simulink model "Xe_Model_Redo_June_26"  (R2018a)
settings: Solver=VariableStepAuto  StartTime=0.0  StopTime=5E5+96*60*60  RelTol=1e-3
values from neighbouring files (symbols this model uses):
  A_pipe = pi*r_pipe^2    (= 0.0126676869774)    [Startup_Script.m]
  alpha_FS = 0.517E-16    (= 5.17e-17)    [Startup_Script.m]
  alpha_G_R1 = 0.334E-17    (= 3.34e-18)    [Startup_Script.m]
  alpha_G_R2 = 0.699E-17    (= 6.99e-18)    [Startup_Script.m]
  alpha_G_R3 = 0.669E-17    (= 6.69e-18)    [Startup_Script.m]
  alpha_G_R4 = 0.791E-18    (= 7.91e-19)    [Startup_Script.m]
  D_g = 2.37E-9    (= 2.37e-09)    [Startup_Script.m]
  epsilon = 0.1    [Startup_Script.m]
  eta_b = 1E-4    (= 0.0001)    [Startup_Script.m]
  eta_fs = 1.2E-4    (= 0.00012)    [Startup_Script.m]
  f_cv = 0.004    [Startup_Script.m]
  FS_Mu_A = 4340    [Startup_Script.m]
  FS_Mu_K = 0.084    [Startup_Script.m]
  FS_Mu_MSRE = 0.007027    [Startup_Script.m]
  FS_rho_A = 3.628    [Startup_Script.m]
  FS_rho_B = 0.00066    [Startup_Script.m]
  FS_rho_MSRE = 2082    [Startup_Script.m]
  gamma_i = 0.0293524    [Startup_Script.m]
  gamma_te = 0.0322482    [Startup_Script.m]
  gamma_xe = 0.00257324    [Startup_Script.m]
  h_fc = 1.6    [Startup_Script.m]
  H_Xe_a = 5.713e-13    [Startup_Script.m]
  H_Xe_b = -7.937e-10    [Startup_Script.m]
  H_Xe_c = 2.809e-07    [Startup_Script.m]
  HX_r_Tube = ((0.5-0.042)/2)*2.54E-2    (= 0.0058166)    [Startup_Script.m]
  HX_XS = HX_N_Tubes*(pi*HX_r_Tube^2)    (= 0.0168999490356)    [Startup_Script.m]
  k_b = 1.3806E-23    (= 1.3806e-23)    [Startup_Script.m]
  lambda_i = 2.9306070546251702E-5    (= 2.93060705463e-05)    [Startup_Script.m]
  lambda_te = 0.036481430555786593    (= 0.0364814305558)    [Startup_Script.m]
  lambda_xe = 2.0924e-05    [Startup_Script.m]
  N_FC_R1 = 12    [Startup_Script.m]
  N_FC_R2 = 940    [Startup_Script.m]
  N_FC_R3 = 108    [Startup_Script.m]
  N_FC_R4 = 78    [Startup_Script.m]
  P_pump = 35420    [Startup_Script.m]
  phi0 = 3.98E+17    (= 3.98e+17)    [Startup_Script.m]
  phi_G_R_1 = mean(interp1(phi_G_R,phi_G_phi, linspace(0,r_g_r1)))    [Startup_Script.m]
  phi_G_R_2 = mean(interp1(phi_G_R,phi_G_phi, linspace(r_g_r1,r_g_r2)))    [Startup_Script.m]
  phi_G_R_3 = mean(interp1(phi_G_R,phi_G_phi, linspace(r_g_r2,r_g_r3)))    [Startup_Script.m]
  phi_G_R_4 = mean(interp1(phi_G_R,phi_G_phi, linspace(r_g_r3,r_g_r4)))    [Startup_Script.m]
  Q_strpr = 0.003155    [Startup_Script.m]
  Q_tot = 0.07571    [Startup_Script.m]
  r_b = 0.000254    [Startup_Script.m]
  r_fc = 0.79e-2    (= 0.0079)    [Startup_Script.m]
  r_pipe = (5E-2*2.54)/2    (= 0.0635)    [Startup_Script.m]
  r_xe = 2.16E-10    (= 2.16e-10)    [Startup_Script.m]
  Re_CA = 25800    [Startup_Script.m]
  Re_LH = 1E4    (= 10000)    [Startup_Script.m]
  Re_UH = 1E4    (= 10000)    [Startup_Script.m]
  sig_a_xe = 1.18E-22    (= 1.18e-22)    [Startup_Script.m]
  Sig_f = 0.15    [Startup_Script.m]
  T_CA_0 = T_INLET    (= 907.594444444)    [Startup_Script.m]
  T_FP_0 = T_OUTLET    (= 935.372222222)    [Startup_Script.m]
  T_FS_R_1_0 = mean(interp1(R_fs_m,T_fs_K, linspace(0,r_g_r1)))    [Startup_Script.m]
  T_FS_R_2_0 = mean(interp1(R_fs_m,T_fs_K, linspace(r_g_r1,r_g_r2)))    [Startup_Script.m]
  T_FS_R_3_0 = mean(interp1(R_fs_m,T_fs_K, linspace(r_g_r2,r_g_r3)))    [Startup_Script.m]
  T_FS_R_4_0 = mean(interp1(R_fs_m,T_fs_K, linspace(r_g_r3,r_g_r4)))    [Startup_Script.m]
  T_G_R_1_0 = mean(interp1(R_gr_m,T_gr_K, linspace(0,r_g_r1)))    [Startup_Script.m]
  T_HX_0 = 0.5*(T_OUTLET + T_INLET)    (= 921.483333333)    [Startup_Script.m]
  T_LH_0 = T_INLET    (= 907.594444444)    [Startup_Script.m]
  T_Mes = 928.15    [Startup_Script.m]
  T_P100_0 = T_OUTLET    (= 935.372222222)    [Startup_Script.m]
  T_P101_0 = T_OUTLET    (= 935.372222222)    [Startup_Script.m]
  T_P102_0 = T_INLET    (= 907.594444444)    [Startup_Script.m]
  T_Salt_0 = 900    [Startup_Script.m]
  T_UH_0 = T_OUTLET    (= 935.372222222)    [Startup_Script.m]
  U_FC_R1 = 0.607    [Startup_Script.m]
  U_FC_R2 = 0.183    [Startup_Script.m]
  U_FC_R3 = 0.454    [Startup_Script.m]
  U_FC_R4 = 0.250    (= 0.25)    [Startup_Script.m]
  V_CA_0 = 9.7*cubed_foot_to_cubed_meter    (= 0.274673445)    [Startup_Script.m]
  V_FP_0 = (0.9+3.2)*cubed_foot_to_cubed_meter    (= 0.116099085)    [Startup_Script.m]
  V_HX_0 = 6.1*cubed_foot_to_cubed_meter    (= 0.172732785)    [Startup_Script.m]
  V_LH_0 = 10.0*cubed_foot_to_cubed_meter    (= 0.2831685)    [Startup_Script.m]
  V_P100_0 = 2.1*cubed_foot_to_cubed_meter    (= 0.059465385)    [Startup_Script.m]
  V_P101_0 = 0.8*cubed_foot_to_cubed_meter    (= 0.02265348)    [Startup_Script.m]
  V_P102_0 = 2.2*cubed_foot_to_cubed_meter    (= 0.06229707)    [Startup_Script.m]
  V_R1_0 = V_Core_FS_0 *N_FC_R1/N_FC_tot    (= 0.00753107712766)    [Startup_Script.m]
  V_R2_0 = V_Core_FS_0 *N_FC_R2/N_FC_tot    (= 0.589934375)    [Startup_Script.m]
  V_R3_0 = V_Core_FS_0 *N_FC_R3/N_FC_tot    (= 0.0677796941489)    [Startup_Script.m]
  V_R4_0 = V_Core_FS_0 *N_FC_R4/N_FC_tot    (= 0.0489520013298)    [Startup_Script.m]
  V_UH_0 = 10.5*cubed_foot_to_cubed_meter    (= 0.297326925)    [Startup_Script.m]
undefined symbols (not defined in the file or in its folder): magnitude, V_CA, V_HX, V_P2, V_P3, V_R1, V_R2, V_R3, V_R4, V_UH
libraries: simulink x4, dspindex x4, dspstat3 x4, SignalEditorBlockLib x2
(part 3 of 11)

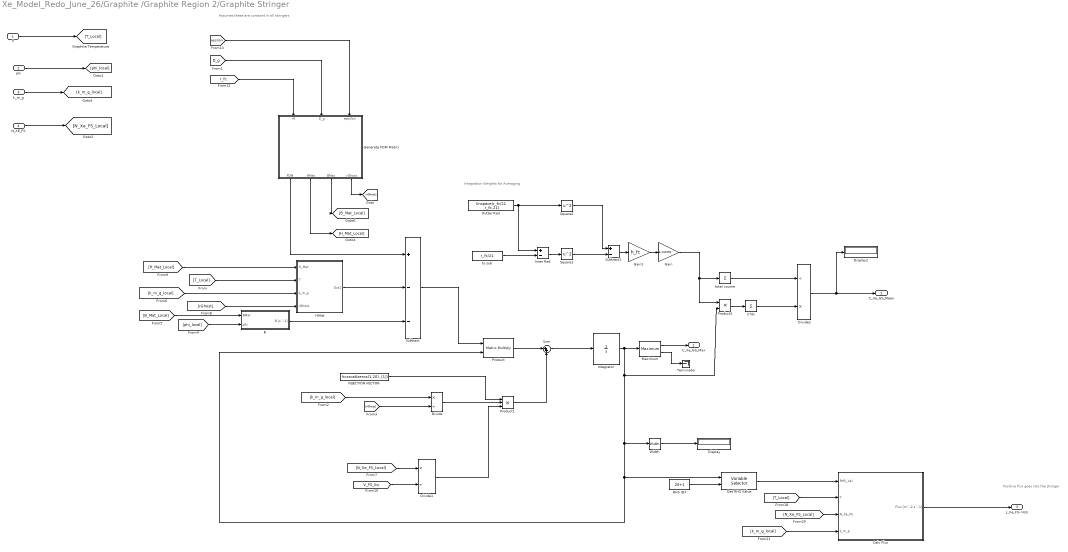
== system Xe_Model_Redo_June_26/Graphite /Graphite Region 2/Graphite Stringer ==
  note: Integration Weights for Averaging
  note: Assumes these are constant in all stringers
  note: Positive flux goes into the stringer
  T : Inport
  phi : Inport  Port=2
  k_m_g : Inport  Port=3
  N_XE_FS : Inport  Port=4
  B : Subsystem
  C*dv : Sum  Inputs=+
  Calc Flux : Subsystem
  Display : Display
  Display2 : Display
  Divide : Product  Inputs=*/
  Divide1 : Product  Inputs=*/
  Divide2 : Product  Inputs=/*
  Gain : Gain  Gain=3.141592
  Gain1 : Gain  Gain=h_fc
  "Generate FDM Matrix " : MATLAB Function  TreatAsAtomicUnit=on
  Get RHS Value : dspindex/Variable Selector  NumInputs=1  rowsOrCols=Rows  IdxMode=Variable  Elements=[1 3]  ZerOneIdxMode=One-based  errmode=Clip Index  FillMode=on  FillValues=0
  HMat : Subsystem
  INJECTION VECTOR : Constant  Value=horzcat(zeros(1,20), [1])
  Inner Rad : Sum  Inputs=+-
  Integrator : Integrator
  Maximum : dspstat3/Maximum  operation=maximum  fcn=Value and Index  indexBase=One  operateOver=Each column  Dimension=1  InputProcessing=Columns as channels (frame based)  reset=None  roiEnable=off  roiType=Rectangles  roiPortion=Entire ROI  roiOutput=Individual statistics for each ROI  roiFlag=off  roundingMode=Floor  overflowMode=off  accumDataTypeStr=Inherit: Same as product output  accumLastDataTypeStr=Inherit: Same as product output
  Outter Rad : Constant  Value=linspace(r_fc/21 ,r_fc,21)
  Product : Product  Multiplication=Matrix(*)
  Product1 : Product  Inputs=3
  Product2 : Product
  RHS IDX : Constant  Value=20+1
  Square1 : Math  Operator=square  SaturateOnIntegerOverflow=on
  Square2 : Math  Operator=square  SaturateOnIntegerOverflow=on
  Subtract : Sum  Inputs=+--
  Subtract1 : Sum  Inputs=+-
  Sum : Sum  Inputs=|++
  Terminator : Terminator
  Width : Width
  to sub : Constant  Value=r_fc/21
  total voume : Sum  Inputs=+
  C_Xe_GS_Max : Outport
  C_Xe_GS_Mean : Outport  Port=2
  J_Xe_FS->GS : Outport  Port=3
  wires:
  Get RHS Value/1 -> Calc Flux/1(RHS_Val)
  Calc Flux/1("Flux [m^-2 s^-1] ") -> J_Xe_FS->GS/1
  HMat/1(Out1) -> Subtract/2
  Maximum/1 -> C_Xe_GS_Max/1
  [rGhost] -> Divide/2
  Divide/1 -> Product1/2
  "Generate FDM Matrix "/1(FDM) -> Subtract/1
  "Generate FDM Matrix "/4(rGhost) -> [rGhost]
  [B_Mat_Local] -> B/1(BMat)
  phi/1 -> [phi_local]
  Subtract/1 -> Product/1
  Divide1/1 -> Product1/3
  Integrator/1 -> Product2/2, Width/1, Product/2, Get RHS Value/1, Maximum/1
  INJECTION VECTOR/1 -> Product1/1
  Product/1 -> Sum/1
  [T_Local] -> HMat/2(T)
  [epsilon] -> "Generate FDM Matrix "/3(epsilon)
  k_m_g/1 -> [k_m_g_local]
  [phi_local] -> B/2(phi)
  [k_m_g_local] -> HMat/3(k_m_g)
  [D_g] -> "Generate FDM Matrix "/2(D_g)
  "Generate FDM Matrix "/3(BMat) -> [B_Mat_Local]
  T/1 -> [T_Local]
  "Generate FDM Matrix "/2(HMat) -> [H_Mat_Local]
  [H_Mat_Local] -> HMat/1(H_Mat)
  [rGhost] -> HMat/4(rGhost)
  [k_m_g_local] -> Divide/1
  [r_fc] -> "Generate FDM Matrix "/1(r0)
  B/1("B [s^-1] ") -> Subtract/3
  Product1/1 -> Sum/2
  Sum/1 -> Integrator/1
  [V_FS_liq] -> Divide1/2
  RHS IDX/1 -> Get RHS Value/2
  [T_Local] -> Calc Flux/2(T)
  N_XE_FS/1 -> [N_Xe_FS_Local]
  [N_Xe_FS_Local] -> Divide1/1
  [k_m_g_local] -> Calc Flux/4(k_m_g)
  [N_Xe_FS_Local] -> Calc Flux/3(N_Xe_FS)
  Width/1 -> Display/1
  Outter Rad/1 -> Inner Rad/1, Square2/1
  Subtract1/1 -> Gain1/1
  Square1/1 -> Subtract1/2
  Square2/1 -> Subtract1/1
  Gain1/1 -> Gain/1
  to sub/1 -> Inner Rad/2
  Inner Rad/1 -> Square1/1
  Gain/1 -> Product2/1, total voume/1
  total voume/1 -> Divide2/1
  Product2/1 -> C*dv/1
  Divide2/1 -> Display2/1, C_Xe_GS_Mean/1
  C*dv/1 -> Divide2/2
  Maximum/2 -> Terminator/1

== system Xe_Model_Redo_June_26/Graphite /Graphite Region 3/Graphite MTC R1 ==
  note: Diemnsionless Numbers
  note: Thermophysical Properties
  T_Salt : Inport
  U_FC [m/s] : Inport  Port=2
  Constant : Constant  Value=0.023
  Constant1 : Constant  Value=0.8
  Constant2 : Constant  Value=0.4
  Density W Scaling : Subsystem
  Display : Display
  Divide : Product  Inputs=*/
  Gain : Gain  Gain=2
  Mass Diffusion Coeffecient [m^2 /s] : Subsystem
  Math Function : Math  Operator=pow  SaturateOnIntegerOverflow=on
  Math Function1 : Math  Operator=pow  SaturateOnIntegerOverflow=on
  Product : Product
  Reynolds Number : Subsystem
  Schmidt Number : Subsystem
  Sherwood Number : Product  Inputs=3
  Viscosity W Scaling : Subsystem
  k_m_g [m/s] : Outport
  wires:
  [D_FS_Local] -> Divide/1
  Constant2/1 -> Math Function1/2
  [r_fc] -> Gain/1
  Constant/1 -> Sherwood Number/1
  Sherwood Number/1 -> Product/1
  [Sc_FC_Local] -> Math Function1/1
  Divide/1 -> Product/2
  Math Function/1 -> Sherwood Number/2
  Constant1/1 -> Math Function/2
  Product/1 -> k_m_g [m/s]/1
  [Re_FC_Local] -> Math Function/1
  Math Function1/1 -> Sherwood Number/3
  Viscosity W Scaling/1(mu [Pa-s]) -> Mass Diffusion Coeffecient [m^2 /s]/1(Mu), [Mu_FS_Local]
  Density W Scaling/1(rho_FS [kg/m^3]) -> [Rho_FS_Local]
  Mass Diffusion Coeffecient [m^2 /s]/1(D [m^2/s]) -> [D_FS_Local]
  T_Salt/1 -> Mass Diffusion Coeffecient [m^2 /s]/2(T_Salt [k]), Density W Scaling/1(T_Salt [k]), Viscosity W Scaling/1(T_Salt [k])
  Schmidt Number/1(Sc) -> [Sc_FC_Local]
  Reynolds Number/1(Re) -> Display/1, [Re_FC_Local]
  U_FC [m/s]/1 -> Reynolds Number/1(Flow_Velocity [m/s])
  [Rho_FS_Local] -> Reynolds Number/2(rho [kg/m^3])
  [Mu_FS_Local] -> Reynolds Number/3(mu [Pa s])
  [Mu_FS_Local] -> Schmidt Number/1(mu [Pa s])
  [Rho_FS_Local] -> Schmidt Number/2(rho [kg/m^3])
  [D_FS_Local] -> Schmidt Number/3(D [m^2/s])
  Gain/1 -> Divide/2

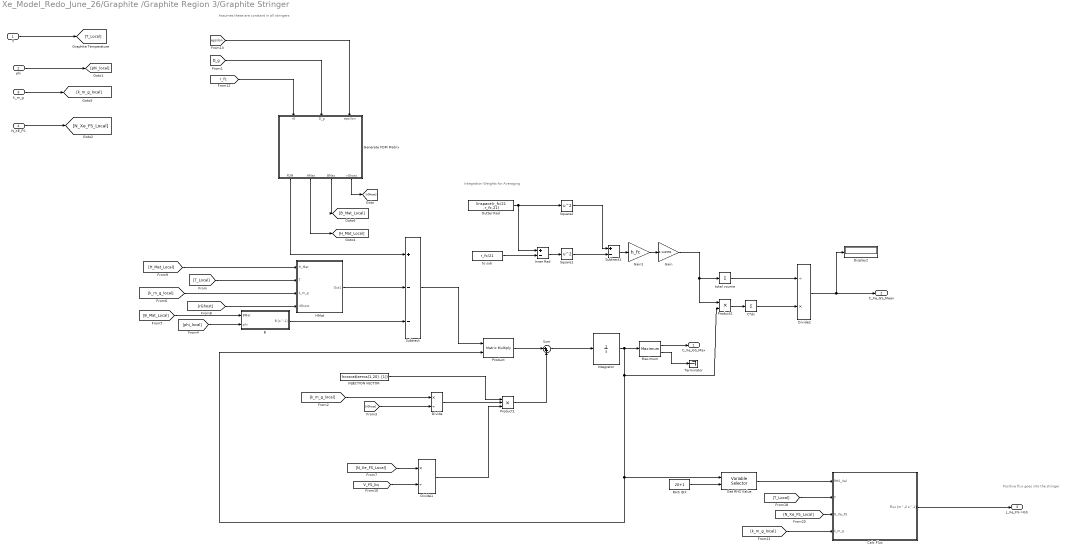
== system Xe_Model_Redo_June_26/Graphite /Graphite Region 3/Graphite Stringer ==
  note: Integration Weights for Averaging
  note: Assumes these are constant in all stringers
  note: Positive flux goes into the stringer
  T : Inport
  phi : Inport  Port=2
  k_m_g : Inport  Port=3
  N_XE_FS : Inport  Port=4
  B : Subsystem
  C*dv : Sum  Inputs=+
  Calc Flux : Subsystem
  Display2 : Display
  Divide : Product  Inputs=*/
  Divide1 : Product  Inputs=*/
  Divide2 : Product  Inputs=/*
  Gain : Gain  Gain=3.141592
  Gain1 : Gain  Gain=h_fc
  "Generate FDM Matrix " : MATLAB Function  TreatAsAtomicUnit=on
  Get RHS Value : dspindex/Variable Selector  NumInputs=1  rowsOrCols=Rows  IdxMode=Variable  Elements=[1 3]  ZerOneIdxMode=One-based  errmode=Clip Index  FillMode=on  FillValues=0
  HMat : Subsystem
  INJECTION VECTOR : Constant  Value=horzcat(zeros(1,20), [1])
  Inner Rad : Sum  Inputs=+-
  Integrator : Integrator
  Maximum : dspstat3/Maximum  operation=maximum  fcn=Value and Index  indexBase=One  operateOver=Each column  Dimension=1  InputProcessing=Columns as channels (frame based)  reset=None  roiEnable=off  roiType=Rectangles  roiPortion=Entire ROI  roiOutput=Individual statistics for each ROI  roiFlag=off  roundingMode=Floor  overflowMode=off  accumDataTypeStr=Inherit: Same as product output  accumLastDataTypeStr=Inherit: Same as product output
  Outter Rad : Constant  Value=linspace(r_fc/21 ,r_fc,21)
  Product : Product  Multiplication=Matrix(*)
  Product1 : Product  Inputs=3
  Product2 : Product
  RHS IDX : Constant  Value=20+1
  Square1 : Math  Operator=square  SaturateOnIntegerOverflow=on
  Square2 : Math  Operator=square  SaturateOnIntegerOverflow=on
  Subtract : Sum  Inputs=+--
  Subtract1 : Sum  Inputs=+-
  Sum : Sum  Inputs=|++
  Terminator : Terminator
  to sub : Constant  Value=r_fc/21
  total voume : Sum  Inputs=+
  C_Xe_GS_Max : Outport
  C_Xe_GS_Mean : Outport  Port=2
  J_Xe_FS->GS : Outport  Port=3
  wires:
  Get RHS Value/1 -> Calc Flux/1(RHS_Val)
  Calc Flux/1("Flux [m^-2 s^-1] ") -> J_Xe_FS->GS/1
  HMat/1(Out1) -> Subtract/2
  Maximum/1 -> C_Xe_GS_Max/1
  [rGhost] -> Divide/2
  Divide/1 -> Product1/2
  "Generate FDM Matrix "/1(FDM) -> Subtract/1
  "Generate FDM Matrix "/4(rGhost) -> [rGhost]
  [B_Mat_Local] -> B/1(BMat)
  phi/1 -> [phi_local]
  Subtract/1 -> Product/1
  Divide1/1 -> Product1/3
  Integrator/1 -> Product2/2, Product/2, Get RHS Value/1, Maximum/1
  INJECTION VECTOR/1 -> Product1/1
  Product/1 -> Sum/1
  [T_Local] -> HMat/2(T)
  [epsilon] -> "Generate FDM Matrix "/3(epsilon)
  k_m_g/1 -> [k_m_g_local]
  [phi_local] -> B/2(phi)
  [k_m_g_local] -> HMat/3(k_m_g)
  [D_g] -> "Generate FDM Matrix "/2(D_g)
  "Generate FDM Matrix "/3(BMat) -> [B_Mat_Local]
  T/1 -> [T_Local]
  "Generate FDM Matrix "/2(HMat) -> [H_Mat_Local]
  [H_Mat_Local] -> HMat/1(H_Mat)
  [rGhost] -> HMat/4(rGhost)
  [k_m_g_local] -> Divide/1
  [r_fc] -> "Generate FDM Matrix "/1(r0)
  B/1("B [s^-1] ") -> Subtract/3
  Product1/1 -> Sum/2
  Sum/1 -> Integrator/1
  [V_FS_liq] -> Divide1/2
  RHS IDX/1 -> Get RHS Value/2
  [T_Local] -> Calc Flux/2(T)
  N_XE_FS/1 -> [N_Xe_FS_Local]
  [N_Xe_FS_Local] -> Divide1/1
  [k_m_g_local] -> Calc Flux/4(k_m_g)
  [N_Xe_FS_Local] -> Calc Flux/3(N_Xe_FS)
  Outter Rad/1 -> Inner Rad/1, Square2/1
  Subtract1/1 -> Gain1/1
  Square1/1 -> Subtract1/2
  Square2/1 -> Subtract1/1
  Gain1/1 -> Gain/1
  to sub/1 -> Inner Rad/2
  Inner Rad/1 -> Square1/1
  Gain/1 -> Product2/1, total voume/1
  total voume/1 -> Divide2/1
  Product2/1 -> C*dv/1
  Divide2/1 -> Display2/1, C_Xe_GS_Mean/1
  C*dv/1 -> Divide2/2
  Maximum/2 -> Terminator/1

== system Xe_Model_Redo_June_26/Graphite /Graphite Region 4/Graphite MTC R1 ==
  note: Diemnsionless Numbers
  note: Thermophysical Properties
  T_Salt : Inport
  U_FC [m/s] : Inport  Port=2
  Constant : Constant  Value=0.023
  Constant1 : Constant  Value=0.8
  Constant2 : Constant  Value=0.4
  Density W Scaling : Subsystem
  Display : Display
  Divide : Product  Inputs=*/
  Gain : Gain  Gain=2
  Mass Diffusion Coeffecient [m^2 /s] : Subsystem
  Math Function : Math  Operator=pow  SaturateOnIntegerOverflow=on
  Math Function1 : Math  Operator=pow  SaturateOnIntegerOverflow=on
  Product : Product
  Reynolds Number : Subsystem
  Schmidt Number : Subsystem
  Sherwood Number : Product  Inputs=3
  Viscosity W Scaling : Subsystem
  k_m_g [m/s] : Outport
  wires:
  [D_FS_Local] -> Divide/1
  Constant2/1 -> Math Function1/2
  [r_fc] -> Gain/1
  Constant/1 -> Sherwood Number/1
  Sherwood Number/1 -> Product/1
  [Sc_FC_Local] -> Math Function1/1
  Divide/1 -> Product/2
  Math Function/1 -> Sherwood Number/2
  Constant1/1 -> Math Function/2
  Product/1 -> k_m_g [m/s]/1
  [Re_FC_Local] -> Math Function/1
  Math Function1/1 -> Sherwood Number/3
  Viscosity W Scaling/1(mu [Pa-s]) -> Mass Diffusion Coeffecient [m^2 /s]/1(Mu), [Mu_FS_Local]
  Density W Scaling/1(rho_FS [kg/m^3]) -> [Rho_FS_Local]
  Mass Diffusion Coeffecient [m^2 /s]/1(D [m^2/s]) -> [D_FS_Local]
  T_Salt/1 -> Mass Diffusion Coeffecient [m^2 /s]/2(T_Salt [k]), Density W Scaling/1(T_Salt [k]), Viscosity W Scaling/1(T_Salt [k])
  Schmidt Number/1(Sc) -> [Sc_FC_Local]
  Reynolds Number/1(Re) -> Display/1, [Re_FC_Local]
  U_FC [m/s]/1 -> Reynolds Number/1(Flow_Velocity [m/s])
  [Rho_FS_Local] -> Reynolds Number/2(rho [kg/m^3])
  [Mu_FS_Local] -> Reynolds Number/3(mu [Pa s])
  [Mu_FS_Local] -> Schmidt Number/1(mu [Pa s])
  [Rho_FS_Local] -> Schmidt Number/2(rho [kg/m^3])
  [D_FS_Local] -> Schmidt Number/3(D [m^2/s])
  Gain/1 -> Divide/2

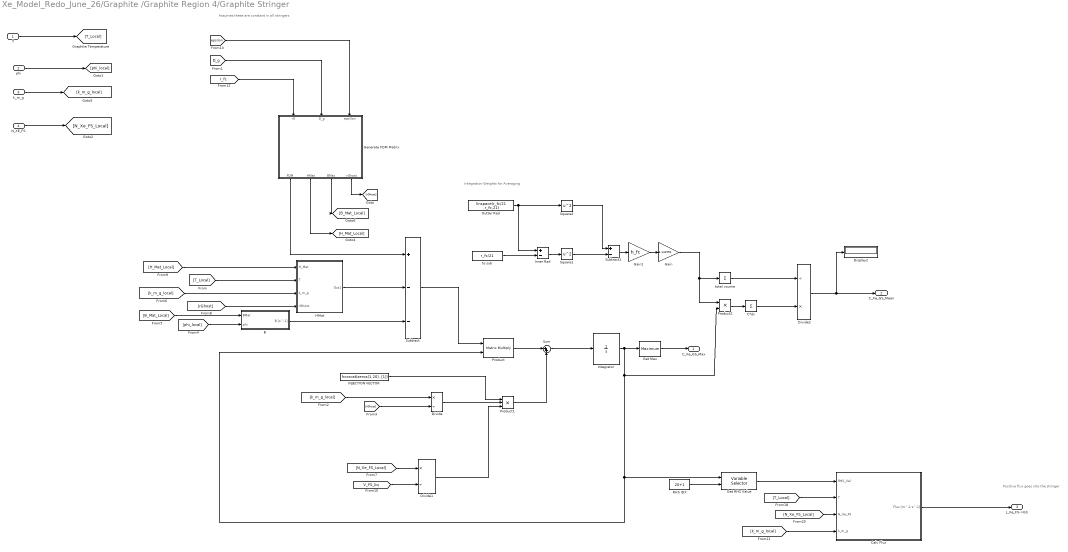
== system Xe_Model_Redo_June_26/Graphite /Graphite Region 4/Graphite Stringer ==
  note: Integration Weights for Averaging
  note: Assumes these are constant in all stringers
  note: Positive flux goes into the stringer
  T : Inport
  phi : Inport  Port=2
  k_m_g : Inport  Port=3
  N_XE_FS : Inport  Port=4
  B : Subsystem
  C*dv : Sum  Inputs=+
  Calc Flux : Subsystem
  Display2 : Display
  Divide : Product  Inputs=*/
  Divide1 : Product  Inputs=*/
  Divide2 : Product  Inputs=/*
  Gain : Gain  Gain=3.141592
  Gain1 : Gain  Gain=h_fc
  "Generate FDM Matrix " : MATLAB Function  TreatAsAtomicUnit=on
  Get Max : dspstat3/Maximum  operation=maximum  fcn=Value  indexBase=One  operateOver=Each column  Dimension=1  InputProcessing=Columns as channels (frame based)  reset=None  roiEnable=off  roiType=Rectangles  roiPortion=Entire ROI  roiOutput=Individual statistics for each ROI  roiFlag=off  roundingMode=Floor  overflowMode=off  accumDataTypeStr=Inherit: Same as product output  accumLastDataTypeStr=Inherit: Same as product output
  Get RHS Value : dspindex/Variable Selector  NumInputs=1  rowsOrCols=Rows  IdxMode=Variable  Elements=[1 3]  ZerOneIdxMode=One-based  errmode=Clip Index  FillMode=on  FillValues=0
  HMat : Subsystem
  INJECTION VECTOR : Constant  Value=horzcat(zeros(1,20), [1])
  Inner Rad : Sum  Inputs=+-
  Integrator : Integrator
  Outter Rad : Constant  Value=linspace(r_fc/21 ,r_fc,21)
  Product : Product  Multiplication=Matrix(*)
  Product1 : Product  Inputs=3
  Product2 : Product
  RHS IDX : Constant  Value=20+1
  Square1 : Math  Operator=square  SaturateOnIntegerOverflow=on
  Square2 : Math  Operator=square  SaturateOnIntegerOverflow=on
  Subtract : Sum  Inputs=+--
  Subtract1 : Sum  Inputs=+-
  Sum : Sum  Inputs=|++
  to sub : Constant  Value=r_fc/21
  total voume : Sum  Inputs=+
  C_Xe_GS_Max : Outport
  C_Xe_GS_Mean : Outport  Port=2
  J_Xe_FS->GS : Outport  Port=3
  wires:
  Get RHS Value/1 -> Calc Flux/1(RHS_Val)
  Calc Flux/1("Flux [m^-2 s^-1] ") -> J_Xe_FS->GS/1
  HMat/1(Out1) -> Subtract/2
  Get Max/1 -> C_Xe_GS_Max/1
  [rGhost] -> Divide/2
  Divide/1 -> Product1/2
  "Generate FDM Matrix "/1(FDM) -> Subtract/1
  "Generate FDM Matrix "/4(rGhost) -> [rGhost]
  [B_Mat_Local] -> B/1(BMat)
  phi/1 -> [phi_local]
  Subtract/1 -> Product/1
  Divide1/1 -> Product1/3
  Integrator/1 -> Product2/2, Product/2, Get RHS Value/1, Get Max/1
  INJECTION VECTOR/1 -> Product1/1
  Product/1 -> Sum/1
  [T_Local] -> HMat/2(T)
  [epsilon] -> "Generate FDM Matrix "/3(epsilon)
  k_m_g/1 -> [k_m_g_local]
  [phi_local] -> B/2(phi)
  [k_m_g_local] -> HMat/3(k_m_g)
  [D_g] -> "Generate FDM Matrix "/2(D_g)
  "Generate FDM Matrix "/3(BMat) -> [B_Mat_Local]
  T/1 -> [T_Local]
  "Generate FDM Matrix "/2(HMat) -> [H_Mat_Local]
  [H_Mat_Local] -> HMat/1(H_Mat)
  [rGhost] -> HMat/4(rGhost)
  [k_m_g_local] -> Divide/1
  [r_fc] -> "Generate FDM Matrix "/1(r0)
  B/1("B [s^-1] ") -> Subtract/3
  Product1/1 -> Sum/2
  Sum/1 -> Integrator/1
  [V_FS_liq] -> Divide1/2
  RHS IDX/1 -> Get RHS Value/2
  [T_Local] -> Calc Flux/2(T)
  N_XE_FS/1 -> [N_Xe_FS_Local]
  [N_Xe_FS_Local] -> Divide1/1
  [k_m_g_local] -> Calc Flux/4(k_m_g)
  [N_Xe_FS_Local] -> Calc Flux/3(N_Xe_FS)
  Outter Rad/1 -> Inner Rad/1, Square2/1
  Subtract1/1 -> Gain1/1
  Square1/1 -> Subtract1/2
  Square2/1 -> Subtract1/1
  Gain1/1 -> Gain/1
  to sub/1 -> Inner Rad/2
  Inner Rad/1 -> Square1/1
  Gain/1 -> Product2/1, total voume/1
  total voume/1 -> Divide2/1
  Product2/1 -> C*dv/1
  Divide2/1 -> Display2/1, C_Xe_GS_Mean/1
  C*dv/1 -> Divide2/2

== system Xe_Model_Redo_June_26/Xenon Stripper/Bubble Stripping/C_B [atoms//m^3] ==
  N_Xe_B : Inport
  Divide : Product  Inputs=*/
  C_Xe_B : Outport
  wires:
  Divide/1 -> C_Xe_B/1
  N_Xe_B/1 -> Divide/1
  [V_CV_Tot] -> Divide/2

== system Xe_Model_Redo_June_26/Bubbles/Bubble Mass Transfer/Bubble Total KMA/HX KMA ==
  CA  CV Area : Subsystem
  Constant : Constant  Value=V_HX
  Constant1 : Constant  Value=HX_r_Tube
  Constant2 : Constant  Value=HX_XS
  Divide : Product  Inputs=*/
  Pipe Buble MTC1 : Subsystem
  Product : Product
  KMA : Outport
  wires:
  Constant1/1 -> Pipe Buble MTC1/3(r)
  Divide/1 -> Pipe Buble MTC1/1(U)
  [Q_tot] -> Divide/1
  Constant2/1 -> Divide/2
  Pipe Buble MTC1/1(k_m_b) -> Product/2
  Product/1 -> KMA/1
  Constant/1 -> CA  CV Area/1(Node Vol.)
  [T_salt] -> CA  CV Area/2(Node T), Pipe Buble MTC1/2(T)
  CA  CV Area/1(A) -> Product/1

== system Xe_Model_Redo_June_26/Bubbles/Bubble Mass Transfer/Bubble Total KMA/KMA FP ==
  CA  CV Area : Subsystem
  Constant : Constant  Value=V_FP_0
  Product : Product
  Pump Bowl MTC1 : Subsystem
  KMA : Outport
  wires:
  Pump Bowl MTC1/1(k_m) -> Product/2
  Product/1 -> KMA/1
  [T_salt] -> CA  CV Area/2(Node T), Pump Bowl MTC1/1(T)
  Constant/1 -> CA  CV Area/1(Node Vol.)
  CA  CV Area/1(A) -> Product/1

== system Xe_Model_Redo_June_26/Bubbles/Bubble Mass Transfer/Bubble Total KMA/KMA_CA ==
  CA  CV Area : Subsystem
  CA  MTC : Subsystem
  Constant : Constant  Value=V_CA
  Product : Product
  KMA : Outport
  wires:
  CA  MTC/1(k_m_b) -> Product/2
  Product/1 -> KMA/1
  [T_salt] -> CA  CV Area/2(Node T), CA  MTC/1(T)
  CA  CV Area/1(A) -> Product/1
  Constant/1 -> CA  CV Area/1(Node Vol.)

== system Xe_Model_Redo_June_26/Bubbles/Bubble Mass Transfer/Bubble Total KMA/KMA_IC ==
  R1 : Subsystem
  R2 : Subsystem
  R3 : Subsystem
  R4 : Subsystem
  Sum1 : Sum  Inputs=++++
  kmA : Outport
  wires:
  Sum1/1 -> kmA/1
  R2/1(kmA) -> Sum1/2
  R4/1(kmA) -> Sum1/4
  R3/1(kmA) -> Sum1/3
  R1/1(kmA) -> Sum1/1

== system Xe_Model_Redo_June_26/Bubbles/Bubble Mass Transfer/Bubble Total KMA/KMA_LH ==
  Constant : Constant  Value=V_CA
  LH  CV Area : Subsystem
  MTC LH : Subsystem
  k_m A : Product
  kmA : Outport
  wires:
  MTC LH/1(k_m_b) -> k_m A/2
  k_m A/1 -> kmA/1
  Constant/1 -> LH  CV Area/1(Node Vol.)
  [T_salt] -> LH  CV Area/2(Node T), MTC LH/1(T)
  LH  CV Area/1(A) -> k_m A/1

== system Xe_Model_Redo_June_26/Bubbles/Bubble Mass Transfer/Bubble Total KMA/KMA_UH ==
  Constant : Constant  Value=V_UH
  MTC UH : Subsystem
  UH CV Area : Subsystem
  k_m A : Product
  kmA : Outport
  wires:
  MTC UH/1(k_m_b) -> k_m A/2
  k_m A/1 -> kmA/1
  Constant/1 -> UH CV Area/1(Node Vol.)
  [T_salt] -> UH CV Area/2(Node T), MTC UH/1(T)
  UH CV Area/1(A) -> k_m A/1

== system Xe_Model_Redo_June_26/Bubbles/Bubble Mass Transfer/Bubble Total KMA/P1 KMA ==
  CA  CV Area : Subsystem
  Constant : Constant  Value=V_CA
  Constant1 : Constant  Value=r_pipe
  Constant2 : Constant  Value=A_pipe
  Divide : Product  Inputs=*/
  Pipe  MTC : Subsystem
  Product : Product
  kma : Outport
  wires:
  Product/1 -> kma/1
  Pipe  MTC/1(k_m_b) -> Product/2
  Divide/1 -> Pipe  MTC/1(U)
  Constant1/1 -> Pipe  MTC/3(r)
  [Q_tot] -> Divide/1
  Constant2/1 -> Divide/2
  Constant/1 -> CA  CV Area/1(Node Vol.)
  [T_salt] -> CA  CV Area/2(Node T), Pipe  MTC/2(T)
  CA  CV Area/1(A) -> Product/1

== system Xe_Model_Redo_June_26/Bubbles/Bubble Mass Transfer/Bubble Total KMA/P2 KMA ==
  Constant : Constant  Value=V_P2
  Constant1 : Constant  Value=r_pipe
  Constant2 : Constant  Value=A_pipe
  Divide : Product  Inputs=*/
  P2  CV Area : Subsystem
  Pipe  MTC : Subsystem
  Product : Product
  kma : Outport
  wires:
  Product/1 -> kma/1
  Pipe  MTC/1(k_m_b) -> Product/2
  Divide/1 -> Pipe  MTC/1(U)
  Constant1/1 -> Pipe  MTC/3(r)
  [Q_tot] -> Divide/1
  Constant2/1 -> Divide/2
  Constant/1 -> P2  CV Area/1(Node Vol.)
  [T_salt] -> P2  CV Area/2(Node T), Pipe  MTC/2(T)
  P2  CV Area/1(A) -> Product/1

== system Xe_Model_Redo_June_26/Bubbles/Bubble Mass Transfer/Bubble Total KMA/P3 KMA ==
  CA  CV Area : Subsystem
  Constant : Constant  Value=V_P3
  Constant1 : Constant  Value=r_pipe
  Constant2 : Constant  Value=A_pipe
  Divide : Product  Inputs=*/
  Pipe  MTC : Subsystem
  Product : Product
  kma : Outport
  wires:
  Product/1 -> kma/1
  Pipe  MTC/1(k_m_b) -> Product/2
  Divide/1 -> Pipe  MTC/1(U)
  Constant1/1 -> Pipe  MTC/3(r)
  [Q_tot] -> Divide/1
  Constant2/1 -> Divide/2
  Constant/1 -> CA  CV Area/1(Node Vol.)
  [T_salt] -> CA  CV Area/2(Node T), Pipe  MTC/2(T)
  CA  CV Area/1(A) -> Product/1

== system Xe_Model_Redo_June_26/Bubbles/Bubble Mass Transfer/CA/Fuel Salt Concentration1 ==
  N_FS : Inport
  divide : Product  Inputs=*/
  C_Xe Liq FS : Outport
  wires:
  divide/1 -> C_Xe Liq FS/1
  N_FS/1 -> divide/1
  [V_FS_liq] -> divide/2

== system Xe_Model_Redo_June_26/Bubbles/Bubble Mass Transfer/CA/HRT*C_B  ==
  N_Xe Gas Phase : Inport
  T Node : Inport  Port=2
  Calc H_Xe : Subsystem
  Divide : Product  Inputs=*/
  Product : Product  Inputs=3
  Product1 : Product
  HRT*(C_Xe in Gas Phase) : Outport
  wires:
  Product/1 -> Product1/1
  Divide/1 -> Product1/2
  Product1/1 -> HRT*(C_Xe in Gas Phase)/1
  N_Xe Gas Phase/1 -> Divide/1
  Calc H_Xe/1(H_Xe [m^-3 Pa^-1]) -> Product/1
  T Node/1 -> Calc H_Xe/1(T_Salt [K]), Product/3
  [R_gas] -> Product/2
  [V_CV_Tot] -> Divide/2

== system Xe_Model_Redo_June_26/Bubbles/Bubble Mass Transfer/CA/KMA_CA ==
  T FS Node : Inport
  V Gas Node : Inport  Port=2
  CA  CV Area : Subsystem
  CA  MTC : Subsystem
  Product : Product
  KMA : Outport
  wires:
  Product/1 -> KMA/1
  T FS Node/1 -> CA  MTC/1(T)
  CA  CV Area/1(A) -> Product/1
  V Gas Node/1 -> CA  CV Area/1(Node Vol.)
  CA  MTC/1(k_m_b) -> Product/2

== system Xe_Model_Redo_June_26/Bubbles/Bubble Mass Transfer/FP/Fuel Salt Concentration1 ==
  N_FS : Inport
  divide : Product  Inputs=*/
  C_Xe Liq FS : Outport
  wires:
  divide/1 -> C_Xe Liq FS/1
  N_FS/1 -> divide/1
  [V_FS_liq] -> divide/2

== system Xe_Model_Redo_June_26/Bubbles/Bubble Mass Transfer/FP/HRT*C_B  ==
  N_Xe Gas Phase : Inport
  T Node : Inport  Port=2
  Calc H_Xe : Subsystem
  Divide : Product  Inputs=*/
  Product : Product  Inputs=3
  Product1 : Product
  HRT*(C_Xe in Gas Phase) : Outport
  wires:
  Product/1 -> Product1/1
  Divide/1 -> Product1/2
  Product1/1 -> HRT*(C_Xe in Gas Phase)/1
  N_Xe Gas Phase/1 -> Divide/1
  Calc H_Xe/1(H_Xe [m^-3 Pa^-1]) -> Product/1
  T Node/1 -> Calc H_Xe/1(T_Salt [K]), Product/3
  [R_gas] -> Product/2
  [V_CV_Tot] -> Divide/2

== system Xe_Model_Redo_June_26/Bubbles/Bubble Mass Transfer/FP/KMA_FP ==
  T FS Node : Inport
  V Gas Node : Inport  Port=2
  CA  CV Area : Subsystem
  Product : Product
  Pump Bowl MTC : Subsystem
  Sum : Sum  Inputs=+++
  KMA : Outport
  wires:
  Pump Bowl MTC/1(k_m) -> Product/2
  Product/1 -> KMA/1
  CA  CV Area/1(A) -> Product/1
  V Gas Node/1 -> CA  CV Area/1(Node Vol.), Sum/1
  T FS Node/1 -> Pump Bowl MTC/2(T)
  Sum/1 -> Pump Bowl MTC/1(V_Node_Tot)
  [V_FP_liq] -> Sum/3
  [V_FP_excess] -> Sum/2

== system Xe_Model_Redo_June_26/Bubbles/Bubble Mass Transfer/G_R1/Fuel Salt Concentration1 ==
  N_FS : Inport
  divide : Product  Inputs=*/
  C_Xe Liq FS : Outport
  wires:
  divide/1 -> C_Xe Liq FS/1
  N_FS/1 -> divide/1
  [V_FS_liq] -> divide/2

== system Xe_Model_Redo_June_26/Bubbles/Bubble Mass Transfer/G_R1/HRT*C_B  ==
  N_Xe Gas Phase : Inport
  T Node : Inport  Port=2
  Calc H_Xe : Subsystem
  Divide : Product  Inputs=*/
  Product : Product  Inputs=3
  Product1 : Product
  HRT*(C_Xe in Gas Phase) : Outport
  wires:
  Product/1 -> Product1/1
  Divide/1 -> Product1/2
  Product1/1 -> HRT*(C_Xe in Gas Phase)/1
  N_Xe Gas Phase/1 -> Divide/1
  Calc H_Xe/1(H_Xe [m^-3 Pa^-1]) -> Product/1
  T Node/1 -> Calc H_Xe/1(T_Salt [K]), Product/3
  [R_gas] -> Product/2
  [V_CV_Tot] -> Divide/2

== system Xe_Model_Redo_June_26/Bubbles/Bubble Mass Transfer/G_R1/KMA_G_R1 ==
  T FS Node : Inport
  V Gas Node : Inport  Port=2
  CA  CV Area : Subsystem
  Pipe Bubble  MTC : Subsystem
  Product : Product
  KMA : Outport
  wires:
  Product/1 -> KMA/1
  CA  CV Area/1(A) -> Product/1
  V Gas Node/1 -> CA  CV Area/1(Node Vol.)
  [U_FC_R1] -> Pipe Bubble  MTC/1(U)
  Pipe Bubble  MTC/1(k_m_b) -> Product/2
  [r_pipe] -> Pipe Bubble  MTC/3(r)
  T FS Node/1 -> Pipe Bubble  MTC/2(T)

== system Xe_Model_Redo_June_26/Bubbles/Bubble Mass Transfer/G_R2/Fuel Salt Concentration1 ==
  N_FS : Inport
  divide : Product  Inputs=*/
  C_Xe Liq FS : Outport
  wires:
  divide/1 -> C_Xe Liq FS/1
  N_FS/1 -> divide/1
  [V_FS_liq] -> divide/2

== system Xe_Model_Redo_June_26/Bubbles/Bubble Mass Transfer/G_R2/HRT*C_B  ==
  N_Xe Gas Phase : Inport
  T Node : Inport  Port=2
  Calc H_Xe : Subsystem
  Divide : Product  Inputs=*/
  Product : Product  Inputs=3
  Product1 : Product
  HRT*(C_Xe in Gas Phase) : Outport
  wires:
  Product/1 -> Product1/1
  Divide/1 -> Product1/2
  Product1/1 -> HRT*(C_Xe in Gas Phase)/1
  N_Xe Gas Phase/1 -> Divide/1
  Calc H_Xe/1(H_Xe [m^-3 Pa^-1]) -> Product/1
  T Node/1 -> Calc H_Xe/1(T_Salt [K]), Product/3
  [R_gas] -> Product/2
  [V_CV_Tot] -> Divide/2

== system Xe_Model_Redo_June_26/Bubbles/Bubble Mass Transfer/G_R2/KMA_G_R1 ==
  T FS Node : Inport
  V Gas Node : Inport  Port=2
  CA  CV Area : Subsystem
  Pipe Bubble  MTC : Subsystem
  Product : Product
  KMA : Outport
  wires:
  Product/1 -> KMA/1
  CA  CV Area/1(A) -> Product/1
  V Gas Node/1 -> CA  CV Area/1(Node Vol.)
  [U_FC_R1] -> Pipe Bubble  MTC/1(U)
  Pipe Bubble  MTC/1(k_m_b) -> Product/2
  [r_pipe] -> Pipe Bubble  MTC/3(r)
  T FS Node/1 -> Pipe Bubble  MTC/2(T)

== system Xe_Model_Redo_June_26/Bubbles/Bubble Mass Transfer/G_R3/Fuel Salt Concentration1 ==
  N_FS : Inport
  divide : Product  Inputs=*/
  C_Xe Liq FS : Outport
  wires:
  divide/1 -> C_Xe Liq FS/1
  N_FS/1 -> divide/1
  [V_FS_liq] -> divide/2

== system Xe_Model_Redo_June_26/Bubbles/Bubble Mass Transfer/G_R3/HRT*C_B  ==
  N_Xe Gas Phase : Inport
  T Node : Inport  Port=2
  Calc H_Xe : Subsystem
  Divide : Product  Inputs=*/
  Product : Product  Inputs=3
  Product1 : Product
  HRT*(C_Xe in Gas Phase) : Outport
  wires:
  Product/1 -> Product1/1
  Divide/1 -> Product1/2
  Product1/1 -> HRT*(C_Xe in Gas Phase)/1
  N_Xe Gas Phase/1 -> Divide/1
  Calc H_Xe/1(H_Xe [m^-3 Pa^-1]) -> Product/1
  T Node/1 -> Calc H_Xe/1(T_Salt [K]), Product/3
  [R_gas] -> Product/2
  [V_CV_Tot] -> Divide/2

== system Xe_Model_Redo_June_26/Bubbles/Bubble Mass Transfer/G_R3/KMA_G_R1 ==
  T FS Node : Inport
  V Gas Node : Inport  Port=2
  CA  CV Area : Subsystem
  Pipe Bubble  MTC : Subsystem
  Product : Product
  KMA : Outport
  wires:
  Product/1 -> KMA/1
  CA  CV Area/1(A) -> Product/1
  V Gas Node/1 -> CA  CV Area/1(Node Vol.)
  [U_FC_R1] -> Pipe Bubble  MTC/1(U)
  Pipe Bubble  MTC/1(k_m_b) -> Product/2
  [r_pipe] -> Pipe Bubble  MTC/3(r)
  T FS Node/1 -> Pipe Bubble  MTC/2(T)

== system Xe_Model_Redo_June_26/Bubbles/Bubble Mass Transfer/G_R4/Fuel Salt Concentration1 ==
  N_FS : Inport
  divide : Product  Inputs=*/
  C_Xe Liq FS : Outport
  wires:
  divide/1 -> C_Xe Liq FS/1
  N_FS/1 -> divide/1
  [V_FS_liq] -> divide/2

== system Xe_Model_Redo_June_26/Bubbles/Bubble Mass Transfer/G_R4/HRT*C_B  ==
  N_Xe Gas Phase : Inport
  T Node : Inport  Port=2
  Calc H_Xe : Subsystem
  Divide : Product  Inputs=*/
  Product : Product  Inputs=3
  Product1 : Product
  HRT*(C_Xe in Gas Phase) : Outport
  wires:
  Product/1 -> Product1/1
  Divide/1 -> Product1/2
  Product1/1 -> HRT*(C_Xe in Gas Phase)/1
  N_Xe Gas Phase/1 -> Divide/1
  Calc H_Xe/1(H_Xe [m^-3 Pa^-1]) -> Product/1
  T Node/1 -> Calc H_Xe/1(T_Salt [K]), Product/3
  [R_gas] -> Product/2
  [V_CV_Tot] -> Divide/2

== system Xe_Model_Redo_June_26/Bubbles/Bubble Mass Transfer/G_R4/KMA_G_R1 ==
  T FS Node : Inport
  V Gas Node : Inport  Port=2
  CA  CV Area : Subsystem
  Pipe Bubble  MTC : Subsystem
  Product : Product
  KMA : Outport
  wires:
  Product/1 -> KMA/1
  CA  CV Area/1(A) -> Product/1
  V Gas Node/1 -> CA  CV Area/1(Node Vol.)
  [U_FC_R1] -> Pipe Bubble  MTC/1(U)
  Pipe Bubble  MTC/1(k_m_b) -> Product/2
  [r_pipe] -> Pipe Bubble  MTC/3(r)
  T FS Node/1 -> Pipe Bubble  MTC/2(T)

== system Xe_Model_Redo_June_26/Bubbles/Bubble Mass Transfer/HX/Fuel Salt Concentration1 ==
  N_FS : Inport
  divide : Product  Inputs=*/
  C_Xe Liq FS : Outport
  wires:
  divide/1 -> C_Xe Liq FS/1
  N_FS/1 -> divide/1
  [V_FS_liq] -> divide/2

== system Xe_Model_Redo_June_26/Bubbles/Bubble Mass Transfer/HX/HRT*C_B  ==
  N_Xe Gas Phase : Inport
  T Node : Inport  Port=2
  Calc H_Xe : Subsystem
  Divide : Product  Inputs=*/
  Product : Product  Inputs=3
  Product1 : Product
  HRT*(C_Xe in Gas Phase) : Outport
  wires:
  Product/1 -> Product1/1
  Divide/1 -> Product1/2
  Product1/1 -> HRT*(C_Xe in Gas Phase)/1
  N_Xe Gas Phase/1 -> Divide/1
  Calc H_Xe/1(H_Xe [m^-3 Pa^-1]) -> Product/1
  T Node/1 -> Calc H_Xe/1(T_Salt [K]), Product/3
  [R_gas] -> Product/2
  [V_CV_Tot] -> Divide/2

== system Xe_Model_Redo_June_26/Bubbles/Bubble Mass Transfer/HX/KMA_HX ==
  T FS Node : Inport
  V Gas Node : Inport  Port=2
  CA  CV Area : Subsystem
  Constant2 : Constant  Value=HX_XS
  Constant3 : Constant  Value=HX_r_Tube
  Divide : Product  Inputs=*/
  Pipe Buble MTC : Subsystem
  Product : Product
  KMA : Outport
  wires:
  Product/1 -> KMA/1
  CA  CV Area/1(A) -> Product/1
  V Gas Node/1 -> CA  CV Area/1(Node Vol.)
  Divide/1 -> Pipe Buble MTC/1(U)
  Pipe Buble MTC/1(k_m_b) -> Product/2
  Constant2/1 -> Divide/2
  [Q_tot] -> Divide/1
  Constant3/1 -> Pipe Buble MTC/3(r)
  T FS Node/1 -> Pipe Buble MTC/2(T)

== system Xe_Model_Redo_June_26/Bubbles/Bubble Mass Transfer/LH/Fuel Salt Concentration1 ==
  N_FS : Inport
  divide : Product  Inputs=*/
  C_Xe Liq FS : Outport
  wires:
  divide/1 -> C_Xe Liq FS/1
  N_FS/1 -> divide/1
  [V_FS_liq] -> divide/2

== system Xe_Model_Redo_June_26/Bubbles/Bubble Mass Transfer/LH/HRT*C_B  ==
  N_Xe Gas Phase : Inport
  T Node : Inport  Port=2
  Calc H_Xe : Subsystem
  Divide : Product  Inputs=*/
  Product : Product  Inputs=3
  Product1 : Product
  HRT*(C_Xe in Gas Phase) : Outport
  wires:
  Product/1 -> Product1/1
  Divide/1 -> Product1/2
  Product1/1 -> HRT*(C_Xe in Gas Phase)/1
  N_Xe Gas Phase/1 -> Divide/1
  Calc H_Xe/1(H_Xe [m^-3 Pa^-1]) -> Product/1
  T Node/1 -> Calc H_Xe/1(T_Salt [K]), Product/3
  [R_gas] -> Product/2
  [V_CV_Tot] -> Divide/2

== system Xe_Model_Redo_June_26/Bubbles/Bubble Mass Transfer/LH/KMA_LH ==
  T FS Node : Inport
  V Gas Node : Inport  Port=2
  CA  CV Area : Subsystem
  MTC LH : Subsystem
  Product : Product
  KMA : Outport
  wires:
  MTC LH/1(k_m_b) -> Product/2
  Product/1 -> KMA/1
  T FS Node/1 -> MTC LH/1(T)
  CA  CV Area/1(A) -> Product/1
  V Gas Node/1 -> CA  CV Area/1(Node Vol.)

== system Xe_Model_Redo_June_26/Bubbles/Bubble Mass Transfer/P100/Fuel Salt Concentration1 ==
  N_FS : Inport
  divide : Product  Inputs=*/
  C_Xe Liq FS : Outport
  wires:
  divide/1 -> C_Xe Liq FS/1
  N_FS/1 -> divide/1
  [V_FS_liq] -> divide/2

== system Xe_Model_Redo_June_26/Bubbles/Bubble Mass Transfer/P100/HRT*C_B  ==
  N_Xe Gas Phase : Inport
  T Node : Inport  Port=2
  Calc H_Xe : Subsystem
  Divide : Product  Inputs=*/
  Product : Product  Inputs=3
  Product1 : Product
  HRT*(C_Xe in Gas Phase) : Outport
  wires:
  Product/1 -> Product1/1
  Divide/1 -> Product1/2
  Product1/1 -> HRT*(C_Xe in Gas Phase)/1
  N_Xe Gas Phase/1 -> Divide/1
  Calc H_Xe/1(H_Xe [m^-3 Pa^-1]) -> Product/1
  T Node/1 -> Calc H_Xe/1(T_Salt [K]), Product/3
  [R_gas] -> Product/2
  [V_CV_Tot] -> Divide/2

== system Xe_Model_Redo_June_26/Bubbles/Bubble Mass Transfer/P100/KMA_P100 ==
  T FS Node : Inport
  V Gas Node : Inport  Port=2
  CA  CV Area : Subsystem
  Constant2 : Constant  Value=A_pipe
  Divide : Product  Inputs=*/
  Pipe Bubble  MTC : Subsystem
  Product : Product
  KMA : Outport
  wires:
  Product/1 -> KMA/1
  CA  CV Area/1(A) -> Product/1
  V Gas Node/1 -> CA  CV Area/1(Node Vol.)
  Divide/1 -> Pipe Bubble  MTC/1(U)
  Pipe Bubble  MTC/1(k_m_b) -> Product/2
  Constant2/1 -> Divide/2
  [r_pipe] -> Pipe Bubble  MTC/3(r)
  T FS Node/1 -> Pipe Bubble  MTC/2(T)
  [Q_tot] -> Divide/1

== system Xe_Model_Redo_June_26/Bubbles/Bubble Mass Transfer/P101/Fuel Salt Concentration1 ==
  N_FS : Inport
  divide : Product  Inputs=*/
  C_Xe Liq FS : Outport
  wires:
  divide/1 -> C_Xe Liq FS/1
  N_FS/1 -> divide/1
  [V_FS_liq] -> divide/2

== system Xe_Model_Redo_June_26/Bubbles/Bubble Mass Transfer/P101/HRT*C_B  ==
  N_Xe Gas Phase : Inport
  T Node : Inport  Port=2
  Calc H_Xe : Subsystem
  Divide : Product  Inputs=*/
  Product : Product  Inputs=3
  Product1 : Product
  HRT*(C_Xe in Gas Phase) : Outport
  wires:
  Product/1 -> Product1/1
  Divide/1 -> Product1/2
  Product1/1 -> HRT*(C_Xe in Gas Phase)/1
  N_Xe Gas Phase/1 -> Divide/1
  Calc H_Xe/1(H_Xe [m^-3 Pa^-1]) -> Product/1
  T Node/1 -> Calc H_Xe/1(T_Salt [K]), Product/3
  [R_gas] -> Product/2
  [V_CV_Tot] -> Divide/2

== system Xe_Model_Redo_June_26/Bubbles/Bubble Mass Transfer/P101/KMA_P101 ==
  T FS Node : Inport
  V Gas Node : Inport  Port=2
  CA  CV Area : Subsystem
  Constant2 : Constant  Value=A_pipe
  Divide : Product  Inputs=*/
  Pipe Bubble  MTC : Subsystem
  Product : Product
  KMA : Outport
  wires:
  Product/1 -> KMA/1
  CA  CV Area/1(A) -> Product/1
  V Gas Node/1 -> CA  CV Area/1(Node Vol.)
  Divide/1 -> Pipe Bubble  MTC/1(U)
  Pipe Bubble  MTC/1(k_m_b) -> Product/2
  Constant2/1 -> Divide/2
  [r_pipe] -> Pipe Bubble  MTC/3(r)
  T FS Node/1 -> Pipe Bubble  MTC/2(T)
  [Q_tot] -> Divide/1

== system Xe_Model_Redo_June_26/Bubbles/Bubble Mass Transfer/P102/Fuel Salt Concentration1 ==
  N_FS : Inport
  divide : Product  Inputs=*/
  C_Xe Liq FS : Outport
  wires:
  divide/1 -> C_Xe Liq FS/1
  N_FS/1 -> divide/1
  [V_FS_liq] -> divide/2

== system Xe_Model_Redo_June_26/Bubbles/Bubble Mass Transfer/P102/HRT*C_B  ==
  N_Xe Gas Phase : Inport
  T Node : Inport  Port=2
  Calc H_Xe : Subsystem
  Divide : Product  Inputs=*/
  Product : Product  Inputs=3
  Product1 : Product
  HRT*(C_Xe in Gas Phase) : Outport
  wires:
  Product/1 -> Product1/1
  Divide/1 -> Product1/2
  Product1/1 -> HRT*(C_Xe in Gas Phase)/1
  N_Xe Gas Phase/1 -> Divide/1
  Calc H_Xe/1(H_Xe [m^-3 Pa^-1]) -> Product/1
  T Node/1 -> Calc H_Xe/1(T_Salt [K]), Product/3
  [R_gas] -> Product/2
  [V_CV_Tot] -> Divide/2

== system Xe_Model_Redo_June_26/Bubbles/Bubble Mass Transfer/P102/KMA_P102 ==
  T FS Node : Inport
  V Gas Node : Inport  Port=2
  CA  CV Area : Subsystem
  Constant2 : Constant  Value=A_pipe
  Divide : Product  Inputs=*/
  Pipe Bubble  MTC : Subsystem
  Product : Product
  KMA : Outport
  wires:
  Product/1 -> KMA/1
  CA  CV Area/1(A) -> Product/1
  V Gas Node/1 -> CA  CV Area/1(Node Vol.)
  Divide/1 -> Pipe Bubble  MTC/1(U)
  Constant2/1 -> Divide/2
  [r_pipe] -> Pipe Bubble  MTC/3(r)
  T FS Node/1 -> Pipe Bubble  MTC/2(T)
  [Q_tot] -> Divide/1
  Pipe Bubble  MTC/1(k_m_b) -> Product/2

== system Xe_Model_Redo_June_26/Bubbles/Bubble Mass Transfer/UH/Fuel Salt Concentration1 ==
  N_FS : Inport
  divide : Product  Inputs=*/
  C_Xe Liq FS : Outport
  wires:
  divide/1 -> C_Xe Liq FS/1
  N_FS/1 -> divide/1
  [V_FS_liq] -> divide/2

== system Xe_Model_Redo_June_26/Bubbles/Bubble Mass Transfer/UH/HRT*C_B  ==
  N_Xe Gas Phase : Inport
  T Node : Inport  Port=2
  Calc H_Xe : Subsystem
  Divide : Product  Inputs=*/
  Product : Product  Inputs=3
  Product1 : Product
  HRT*(C_Xe in Gas Phase) : Outport
  wires:
  Product/1 -> Product1/1
  Divide/1 -> Product1/2
  Product1/1 -> HRT*(C_Xe in Gas Phase)/1
  N_Xe Gas Phase/1 -> Divide/1
  Calc H_Xe/1(H_Xe [m^-3 Pa^-1]) -> Product/1
  T Node/1 -> Calc H_Xe/1(T_Salt [K]), Product/3
  [R_gas] -> Product/2
  [V_CV_Tot] -> Divide/2

== system Xe_Model_Redo_June_26/Bubbles/Bubble Mass Transfer/UH/KMA_UH ==
  T FS Node : Inport
  V Gas Node : Inport  Port=2
  CA  CV Area : Subsystem
  MTC UH : Subsystem
  Product : Product
  KMA : Outport
  wires:
  MTC UH/1(k_m_b) -> Product/2
  Product/1 -> KMA/1
  T FS Node/1 -> MTC UH/1(T)
  CA  CV Area/1(A) -> Product/1
  V Gas Node/1 -> CA  CV Area/1(Node Vol.)

== system Xe_Model_Redo_June_26/CONSTANTS/V CA/Current Density/Cantor F1 Density ==
  note: K -> deg. C
  T_Salt [k] : Inport
  Constant : Constant  Value=FS_rho_A
  Constant1 : Constant  Value=FS_rho_B
  Constant2 : Constant  Value=273.15
  Display : Display
      settings: Format=short_e
  Display1 : Display
  Product : Product
  Sum : Sum  Inputs=|+-
  Sum1 : Sum  Inputs=+-
  "g/cm^3 -> kg/m^3" : Gain  Gain=1000
  rho [kg/m^3] : Outport
  wires:
  Sum/1 -> "g/cm^3 -> kg/m^3"/1
  Product/1 -> Sum/2
  Constant1/1 -> Display/1, Product/1
  "g/cm^3 -> kg/m^3"/1 -> rho [kg/m^3]/1
  Constant/1 -> Display1/1, Sum/1
  T_Salt [k]/1 -> Sum1/1
  Constant2/1 -> Sum1/2
  Sum1/1 -> Product/2

== system Xe_Model_Redo_June_26/CONSTANTS/V CA/Current Density/Cantor F1 Density1 ==
  note: K -> deg. C
  T_Salt [k] : Inport
  Constant : Constant  Value=FS_rho_A
  Constant1 : Constant  Value=FS_rho_B
  Constant2 : Constant  Value=273.15
  Display : Display
      settings: Format=short_e
  Display1 : Display
  Product : Product
  Sum : Sum  Inputs=|+-
  Sum1 : Sum  Inputs=+-
  "g/cm^3 -> kg/m^3" : Gain  Gain=1000
  rho [kg/m^3] : Outport
  wires:
  Sum/1 -> "g/cm^3 -> kg/m^3"/1
  Product/1 -> Sum/2
  Constant1/1 -> Display/1, Product/1
  "g/cm^3 -> kg/m^3"/1 -> rho [kg/m^3]/1
  Constant/1 -> Display1/1, Sum/1
  T_Salt [k]/1 -> Sum1/1
  Constant2/1 -> Sum1/2
  Sum1/1 -> Product/2

== system Xe_Model_Redo_June_26/CONSTANTS/V CA/Reference Density/Cantor F1 Density ==
  note: K -> deg. C
  T_Salt [k] : Inport
  Constant : Constant  Value=FS_rho_A
  Constant1 : Constant  Value=FS_rho_B
  Constant2 : Constant  Value=273.15
  Display : Display
      settings: Format=short_e
  Display1 : Display
  Product : Product
  Sum : Sum  Inputs=|+-
  Sum1 : Sum  Inputs=+-
  "g/cm^3 -> kg/m^3" : Gain  Gain=1000
  rho [kg/m^3] : Outport
  wires:
  Sum/1 -> "g/cm^3 -> kg/m^3"/1
  Product/1 -> Sum/2
  Constant1/1 -> Display/1, Product/1
  "g/cm^3 -> kg/m^3"/1 -> rho [kg/m^3]/1
  Constant/1 -> Display1/1, Sum/1
  T_Salt [k]/1 -> Sum1/1
  Constant2/1 -> Sum1/2
  Sum1/1 -> Product/2

== system Xe_Model_Redo_June_26/CONSTANTS/V CA/Reference Density/Cantor F1 Density1 ==
  note: K -> deg. C
  T_Salt [k] : Inport
  Constant : Constant  Value=FS_rho_A
  Constant1 : Constant  Value=FS_rho_B
  Constant2 : Constant  Value=273.15
  Display : Display
      settings: Format=short_e
  Display1 : Display
  Product : Product
  Sum : Sum  Inputs=|+-
  Sum1 : Sum  Inputs=+-
  "g/cm^3 -> kg/m^3" : Gain  Gain=1000
  rho [kg/m^3] : Outport
  wires:
  Sum/1 -> "g/cm^3 -> kg/m^3"/1
  Product/1 -> Sum/2
  Constant1/1 -> Display/1, Product/1
  "g/cm^3 -> kg/m^3"/1 -> rho [kg/m^3]/1
  Constant/1 -> Display1/1, Sum/1
  T_Salt [k]/1 -> Sum1/1
  Constant2/1 -> Sum1/2
  Sum1/1 -> Product/2

== system Xe_Model_Redo_June_26/CONSTANTS/V FP/Current Density/Cantor F1 Density ==
  note: K -> deg. C
  T_Salt [k] : Inport
  Constant : Constant  Value=FS_rho_A
  Constant1 : Constant  Value=FS_rho_B
  Constant2 : Constant  Value=273.15
  Display : Display
      settings: Format=short_e
  Display1 : Display
  Product : Product
  Sum : Sum  Inputs=|+-
  Sum1 : Sum  Inputs=+-
  "g/cm^3 -> kg/m^3" : Gain  Gain=1000
  rho [kg/m^3] : Outport
  wires:
  Sum/1 -> "g/cm^3 -> kg/m^3"/1
  Product/1 -> Sum/2
  Constant1/1 -> Display/1, Product/1
  "g/cm^3 -> kg/m^3"/1 -> rho [kg/m^3]/1
  Constant/1 -> Display1/1, Sum/1
  T_Salt [k]/1 -> Sum1/1
  Constant2/1 -> Sum1/2
  Sum1/1 -> Product/2

== system Xe_Model_Redo_June_26/CONSTANTS/V FP/Current Density/Cantor F1 Density1 ==
  note: K -> deg. C
  T_Salt [k] : Inport
  Constant : Constant  Value=FS_rho_A
  Constant1 : Constant  Value=FS_rho_B
  Constant2 : Constant  Value=273.15
  Display : Display
      settings: Format=short_e
  Display1 : Display
  Product : Product
  Sum : Sum  Inputs=|+-
  Sum1 : Sum  Inputs=+-
  "g/cm^3 -> kg/m^3" : Gain  Gain=1000
  rho [kg/m^3] : Outport
  wires:
  Sum/1 -> "g/cm^3 -> kg/m^3"/1
  Product/1 -> Sum/2
  Constant1/1 -> Display/1, Product/1
  "g/cm^3 -> kg/m^3"/1 -> rho [kg/m^3]/1
  Constant/1 -> Display1/1, Sum/1
  T_Salt [k]/1 -> Sum1/1
  Constant2/1 -> Sum1/2
  Sum1/1 -> Product/2

== system Xe_Model_Redo_June_26/CONSTANTS/V FP/Reference Density/Cantor F1 Density ==
  note: K -> deg. C
  T_Salt [k] : Inport
  Constant : Constant  Value=FS_rho_A
  Constant1 : Constant  Value=FS_rho_B
  Constant2 : Constant  Value=273.15
  Display : Display
      settings: Format=short_e
  Display1 : Display
  Product : Product
  Sum : Sum  Inputs=|+-
  Sum1 : Sum  Inputs=+-
  "g/cm^3 -> kg/m^3" : Gain  Gain=1000
  rho [kg/m^3] : Outport
  wires:
  Sum/1 -> "g/cm^3 -> kg/m^3"/1
  Product/1 -> Sum/2
  Constant1/1 -> Display/1, Product/1
  "g/cm^3 -> kg/m^3"/1 -> rho [kg/m^3]/1
  Constant/1 -> Display1/1, Sum/1
  T_Salt [k]/1 -> Sum1/1
  Constant2/1 -> Sum1/2
  Sum1/1 -> Product/2

== system Xe_Model_Redo_June_26/CONSTANTS/V FP/Reference Density/Cantor F1 Density1 ==
  note: K -> deg. C
  T_Salt [k] : Inport
  Constant : Constant  Value=FS_rho_A
  Constant1 : Constant  Value=FS_rho_B
  Constant2 : Constant  Value=273.15
  Display : Display
      settings: Format=short_e
  Display1 : Display
  Product : Product
  Sum : Sum  Inputs=|+-
  Sum1 : Sum  Inputs=+-
  "g/cm^3 -> kg/m^3" : Gain  Gain=1000
  rho [kg/m^3] : Outport
  wires:
  Sum/1 -> "g/cm^3 -> kg/m^3"/1
  Product/1 -> Sum/2
  Constant1/1 -> Display/1, Product/1
  "g/cm^3 -> kg/m^3"/1 -> rho [kg/m^3]/1
  Constant/1 -> Display1/1, Sum/1
  T_Salt [k]/1 -> Sum1/1
  Constant2/1 -> Sum1/2
  Sum1/1 -> Product/2

== system Xe_Model_Redo_June_26/CONSTANTS/V FP1/Current Density/Cantor F1 Density ==
  note: K -> deg. C
  T_Salt [k] : Inport
  Constant : Constant  Value=FS_rho_A
  Constant1 : Constant  Value=FS_rho_B
  Constant2 : Constant  Value=273.15
  Display : Display
      settings: Format=short_e
  Display1 : Display
  Product : Product
  Sum : Sum  Inputs=|+-
  Sum1 : Sum  Inputs=+-
  "g/cm^3 -> kg/m^3" : Gain  Gain=1000
  rho [kg/m^3] : Outport
  wires:
  Sum/1 -> "g/cm^3 -> kg/m^3"/1
  Product/1 -> Sum/2
  Constant1/1 -> Display/1, Product/1
  "g/cm^3 -> kg/m^3"/1 -> rho [kg/m^3]/1
  Constant/1 -> Display1/1, Sum/1
  T_Salt [k]/1 -> Sum1/1
  Constant2/1 -> Sum1/2
  Sum1/1 -> Product/2

== system Xe_Model_Redo_June_26/CONSTANTS/V FP1/Current Density/Cantor F1 Density1 ==
  note: K -> deg. C
  T_Salt [k] : Inport
  Constant : Constant  Value=FS_rho_A
  Constant1 : Constant  Value=FS_rho_B
  Constant2 : Constant  Value=273.15
  Display : Display
      settings: Format=short_e
  Display1 : Display
  Product : Product
  Sum : Sum  Inputs=|+-
  Sum1 : Sum  Inputs=+-
  "g/cm^3 -> kg/m^3" : Gain  Gain=1000
  rho [kg/m^3] : Outport
  wires:
  Sum/1 -> "g/cm^3 -> kg/m^3"/1
  Product/1 -> Sum/2
  Constant1/1 -> Display/1, Product/1
  "g/cm^3 -> kg/m^3"/1 -> rho [kg/m^3]/1
  Constant/1 -> Display1/1, Sum/1
  T_Salt [k]/1 -> Sum1/1
  Constant2/1 -> Sum1/2
  Sum1/1 -> Product/2

== system Xe_Model_Redo_June_26/CONSTANTS/V FP1/Reference Density/Cantor F1 Density ==
  note: K -> deg. C
  T_Salt [k] : Inport
  Constant : Constant  Value=FS_rho_A
  Constant1 : Constant  Value=FS_rho_B
  Constant2 : Constant  Value=273.15
  Display : Display
      settings: Format=short_e
  Display1 : Display
  Product : Product
  Sum : Sum  Inputs=|+-
  Sum1 : Sum  Inputs=+-
  "g/cm^3 -> kg/m^3" : Gain  Gain=1000
  rho [kg/m^3] : Outport
  wires:
  Sum/1 -> "g/cm^3 -> kg/m^3"/1
  Product/1 -> Sum/2
  Constant1/1 -> Display/1, Product/1
  "g/cm^3 -> kg/m^3"/1 -> rho [kg/m^3]/1
  Constant/1 -> Display1/1, Sum/1
  T_Salt [k]/1 -> Sum1/1
  Constant2/1 -> Sum1/2
  Sum1/1 -> Product/2

== system Xe_Model_Redo_June_26/CONSTANTS/V FP1/Reference Density/Cantor F1 Density1 ==
  note: K -> deg. C
  T_Salt [k] : Inport
  Constant : Constant  Value=FS_rho_A
  Constant1 : Constant  Value=FS_rho_B
  Constant2 : Constant  Value=273.15
  Display : Display
      settings: Format=short_e
  Display1 : Display
  Product : Product
  Sum : Sum  Inputs=|+-
  Sum1 : Sum  Inputs=+-
  "g/cm^3 -> kg/m^3" : Gain  Gain=1000
  rho [kg/m^3] : Outport
  wires:
  Sum/1 -> "g/cm^3 -> kg/m^3"/1
  Product/1 -> Sum/2
  Constant1/1 -> Display/1, Product/1
  "g/cm^3 -> kg/m^3"/1 -> rho [kg/m^3]/1
  Constant/1 -> Display1/1, Sum/1
  T_Salt [k]/1 -> Sum1/1
  Constant2/1 -> Sum1/2
  Sum1/1 -> Product/2

== system Xe_Model_Redo_June_26/CONSTANTS/V HX/Current Density/Cantor F1 Density ==
  note: K -> deg. C
  T_Salt [k] : Inport
  Constant : Constant  Value=FS_rho_A
  Constant1 : Constant  Value=FS_rho_B
  Constant2 : Constant  Value=273.15
  Display : Display
      settings: Format=short_e
  Display1 : Display
  Product : Product
  Sum : Sum  Inputs=|+-
  Sum1 : Sum  Inputs=+-
  "g/cm^3 -> kg/m^3" : Gain  Gain=1000
  rho [kg/m^3] : Outport
  wires:
  Sum/1 -> "g/cm^3 -> kg/m^3"/1
  Product/1 -> Sum/2
  Constant1/1 -> Display/1, Product/1
  "g/cm^3 -> kg/m^3"/1 -> rho [kg/m^3]/1
  Constant/1 -> Display1/1, Sum/1
  T_Salt [k]/1 -> Sum1/1
  Constant2/1 -> Sum1/2
  Sum1/1 -> Product/2

== system Xe_Model_Redo_June_26/CONSTANTS/V HX/Current Density/Cantor F1 Density1 ==
  note: K -> deg. C
  T_Salt [k] : Inport
  Constant : Constant  Value=FS_rho_A
  Constant1 : Constant  Value=FS_rho_B
  Constant2 : Constant  Value=273.15
  Display : Display
      settings: Format=short_e
  Display1 : Display
  Product : Product
  Sum : Sum  Inputs=|+-
  Sum1 : Sum  Inputs=+-
  "g/cm^3 -> kg/m^3" : Gain  Gain=1000
  rho [kg/m^3] : Outport
  wires:
  Sum/1 -> "g/cm^3 -> kg/m^3"/1
  Product/1 -> Sum/2
  Constant1/1 -> Display/1, Product/1
  "g/cm^3 -> kg/m^3"/1 -> rho [kg/m^3]/1
  Constant/1 -> Display1/1, Sum/1
  T_Salt [k]/1 -> Sum1/1
  Constant2/1 -> Sum1/2
  Sum1/1 -> Product/2
